simulink model "Lab01"  (R2019a)
settings: Solver=VariableStepAuto  StartTime=0.0  StopTime=8  RelTol=1e-3
settings Model: Creator=Huyco  LastModifiedBy=Huyco

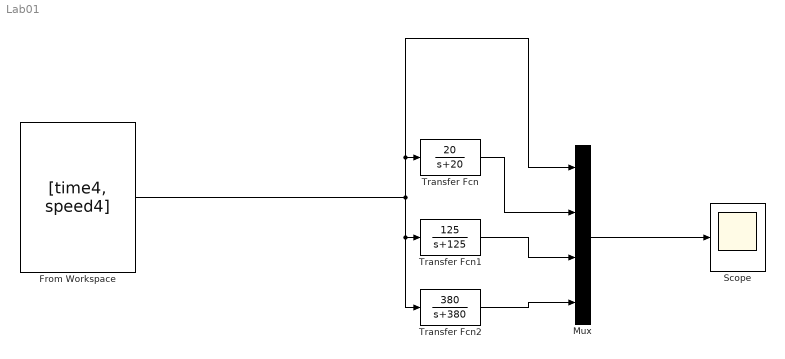
== system Lab01 ==
  From Workspace : FromWorkspace  VariableName=[time4, speed4]  SampleTime=0
  Mux : Mux
  Scope : Scope
  Transfer Fcn : TransferFcn  Numerator=[20]  Denominator=[1 20]
  Transfer Fcn1 : TransferFcn  Numerator=[125]  Denominator=[1 125]
  Transfer Fcn2 : TransferFcn  Numerator=[380]  Denominator=[1 380]
  wires:
  From Workspace/1 -> Mux/1, Transfer Fcn/1, Transfer Fcn1/1, Transfer Fcn2/1
  Transfer Fcn/1 -> Mux/2
  Transfer Fcn1/1 -> Mux/3
  Transfer Fcn2/1 -> Mux/4
  Mux/1 -> Scope/1
